simulink subsystem "WinchControl"  (R2022b)
settings: Solver=VariableStepAuto  StartTime=0.0  StopTime=10.0  RelTol=1e-3
undefined symbols (not defined in the file or in its folder): constr, DiscIntNeverNeededParam, params, winchParameter
libraries: simulink x5, slpidlib x1
settings Model: Creator=dylaneijkelhof  LastModifiedBy=jesse
settings SolverCC: AlgebraicLoopSolver=TrustRegion
settings DebuggingCC: UnconnectedInputMsg=warning  UnconnectedOutputMsg=warning  UnconnectedLineMsg=warning  SFMachineParentedDataDiag=warning
settings ModelReferenceCC: EnableRefExpFcnMdlSchedulingChecks=on

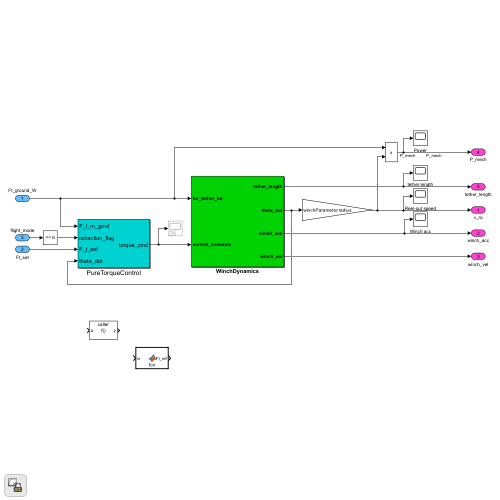
[thumbnail: Simulink's stored preview of the top-level diagram]
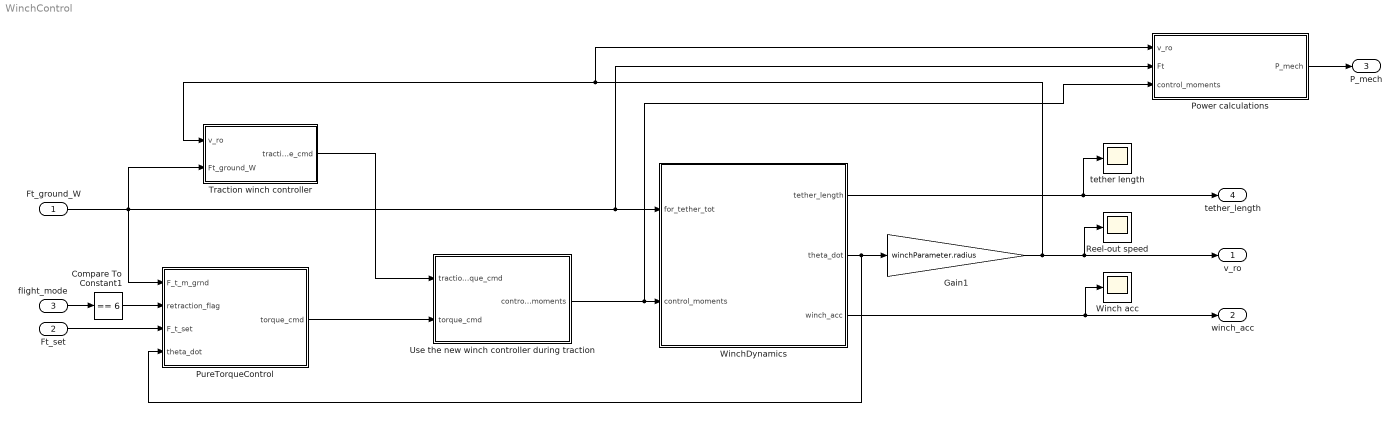
== system WinchControl ==
  Ft_ground_W : Inport  OutDataTypeStr=double  PortDimensions=1
  Ft_set : Inport  Port=2  OutDataTypeStr=double  PortDimensions=1
  flight_mode : Inport  Port=3  OutDataTypeStr=double  PortDimensions=1
  Compare To Constant1 : simulink/Logic and Bit Operations/Compare To Constant  relop===  const=6  OutDataTypeStr=boolean
  Gain1 : Gain  Gain=winchParameter.radius
  Power calculations : Subsystem
  PureTorqueControl : Subsystem
  Reel-out speed : Scope
  Traction winch controller : Subsystem
  Use the new winch controller during traction : Subsystem
  Winch acc : Scope
  WinchDynamics : Subsystem
  tether length : Scope
  v_ro : Outport  OutDataTypeStr=double  PortDimensions=1  VectorParamsAs1DForOutWhenUnconnected=off
  winch_acc : Outport  Port=2  OutDataTypeStr=double  PortDimensions=1  VectorParamsAs1DForOutWhenUnconnected=off
  P_mech : Outport  Port=3  OutDataTypeStr=double  PortDimensions=1  VectorParamsAs1DForOutWhenUnconnected=off
  tether_length : Outport  Port=4  OutDataTypeStr=double  PortDimensions=1  VectorParamsAs1DForOutWhenUnconnected=off
  wires:
  Compare To Constant1/1 -> PureTorqueControl/2(retraction_flag)
  WinchDynamics/1(tether_length) -> tether_length/1, tether length/1
  WinchDynamics/3(winch_acc) -> winch_acc/1, Winch acc/1
  flight_mode/1 -> Compare To Constant1/1
  Ft_set/1 -> PureTorqueControl/3(F_t_set)
  Ft_ground_W/1 -> Power calculations/2(Ft), WinchDynamics/1(for_tether_tot), PureTorqueControl/1(F_t_m_grnd), Traction winch controller/2(Ft_ground_W)
  WinchDynamics/2(theta_dot) -> PureTorqueControl/4(theta_dot), Gain1/1
  Gain1/1 -> Traction winch controller/1(v_ro), Power calculations/1(v_ro), v_ro/1, Reel-out speed/1
  Use the new winch controller during traction/1(control_moments) -> WinchDynamics/2(control_moments), Power calculations/3(control_moments)
  Traction winch controller/1(traction_torque_cmd) -> Use the new winch controller during traction/1(traction_torque_cmd)
  Power calculations/1(P_mech) -> P_mech/1
  PureTorqueControl/1(torque_cmd) -> Use the new winch controller during traction/2(torque_cmd)

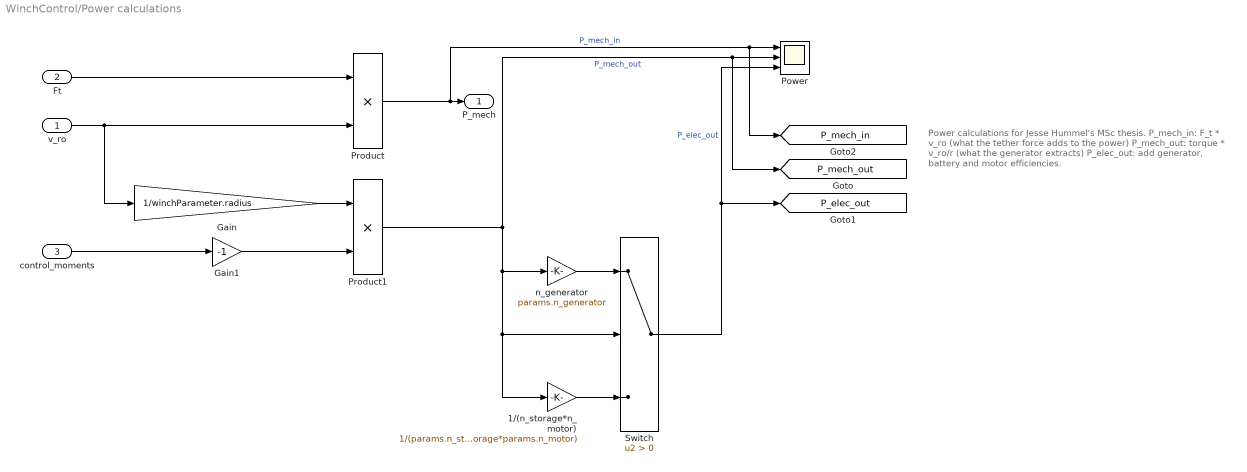
== system WinchControl/Power calculations ==
  note: Power calculations for Jesse Hummel's MSc thesis.
      | P_mech_in: F_t * v_ro (what the tether force adds to the power)
      | P_mech_out: torque * v_ro/r (what the generator extracts)
      | P_elec_out: add generator, battery and motor efficiencies.
  v_ro : Inport
  Ft : Inport  Port=2
  control_moments : Inport  Port=3
  1/(n_storage*n_motor) : Gain  Gain=1/(params.n_storage*params.n_motor)
  Gain : Gain  Gain=1/winchParameter.radius
  Gain1 : Gain  Gain=-1
  Power : Scope  NumInputPorts=3
  Product : Product
  Product1 : Product
  Switch : Switch  Criteria=u2 > Threshold  SaturateOnIntegerOverflow=off  InputSameDT=off
  n_generator : Gain  Gain=params.n_generator
  P_mech : Outport
  tag scope: P_elec_out=global, P_mech_in=global, P_mech_out=global
  wires:
  Gain1/1 -> Product1/2
  Switch/1 -> Power/3, [P_elec_out]  "P_elec_out"
  1/(n_storage*n_motor)/1 -> Switch/3
  n_generator/1 -> Switch/1
  Product1/1 -> Power/2, [P_mech_out], 1/(n_storage*n_motor)/1, Switch/2, n_generator/1  "P_mech_out"
  control_moments/1 -> Gain1/1
  Gain/1 -> Product1/1
  v_ro/1 -> Product/2, Gain/1
  Ft/1 -> Product/1
  Product/1 -> P_mech/1, Power/1, [P_mech_in]  "P_mech_in"

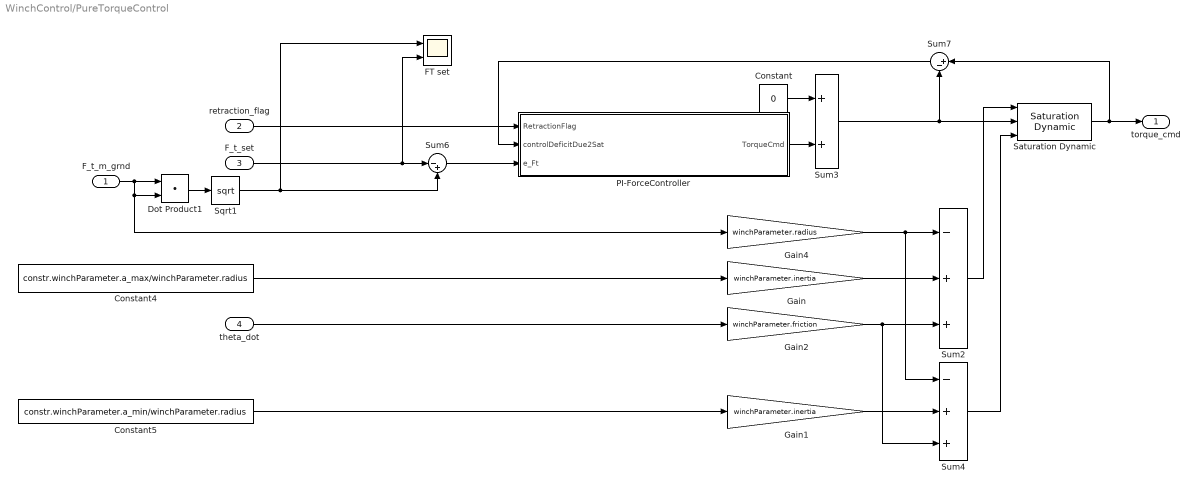
== system WinchControl/PureTorqueControl ==
  F_t_m_grnd : Inport
  retraction_flag : Inport  Port=2
  F_t_set : Inport  Port=3
  theta_dot : Inport  Port=4
  Constant : Constant  Value=0
  Constant4 : Constant  Value=constr.winchParameter.a_max/winchParameter.radius
  Constant5 : Constant  Value=constr.winchParameter.a_min/winchParameter.radius
  Dot Product1 : DotProduct  OutDataTypeStr=Inherit: Inherit via internal rule
  FT set : Scope  NumInputPorts=2
  Gain : Gain  Gain=winchParameter.inertia
  Gain1 : Gain  Gain=winchParameter.inertia
  Gain2 : Gain  Gain=winchParameter.friction
  Gain4 : Gain  Gain=winchParameter.radius
  PI-ForceController : Subsystem
  Saturation Dynamic : simulink/Discontinuities/Saturation Dynamic  OutMin=[]  OutMax=[]  OutDataTypeStr=Inherit: Same as second input  OutDataType=fixdt(1, 16)  OutScaling=2^-10  DoSatur=off
  Sqrt1 : Sqrt
  Sum2 : Sum  Inputs=-++
  Sum3 : Sum
  Sum4 : Sum  Inputs=-++
  Sum6 : Sum  Inputs=|-+
  Sum7 : Sum  Inputs=|+-
  torque_cmd : Outport  VectorParamsAs1DForOutWhenUnconnected=off
  wires:
  Saturation Dynamic/1 -> Sum7/1, torque_cmd/1
  PI-ForceController/1(TorqueCmd) -> Sum3/2
  Sum6/1 -> PI-ForceController/3(e_Ft)
  Sum7/1 -> PI-ForceController/2(controlDeficitDue2Sat)
  theta_dot/1 -> Gain2/1
  F_t_m_grnd/1 -> Gain4/1, Dot Product1/2, Dot Product1/1
  Dot Product1/1 -> Sqrt1/1
  Gain2/1 -> Sum2/3, Sum4/3
  Sum3/1 -> Sum7/2, Saturation Dynamic/2
  Sum4/1 -> Saturation Dynamic/3
  Gain1/1 -> Sum4/2
  Constant5/1 -> Gain1/1
  Sum2/1 -> Saturation Dynamic/1
  Gain/1 -> Sum2/2
  Constant4/1 -> Gain/1
  Gain4/1 -> Sum4/1, Sum2/1
  F_t_set/1 -> Sum6/1, FT set/2
  Constant/1 -> Sum3/1
  retraction_flag/1 -> PI-ForceController/1(RetractionFlag)
  Sqrt1/1 -> Sum6/2, FT set/1

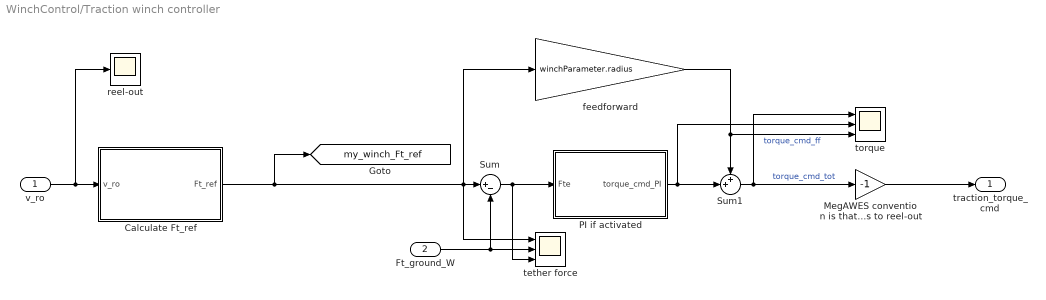
== system WinchControl/Traction winch controller ==
  v_ro : Inport
  Ft_ground_W : Inport  Port=2
  Calculate Ft_ref : Subsystem
  MegAWES convention is that a positive torque leads to reel-out : Gain  Gain=-1
  PI if activated : Subsystem
  Sum : Sum  Inputs=|+-
  Sum1 : Sum  Inputs=++|
  feedforward : Gain  Gain=winchParameter.radius
  reel-out : Scope
  tether force : Scope  NumInputPorts=3
  torque : Scope  NumInputPorts=3
  traction_torque_cmd : Outport
  tag scope: my_winch_Ft_ref=global
  wires:
  PI if activated/1(torque_cmd_PI) -> torque/2, Sum1/2
  Calculate Ft_ref/1(Ft_ref) -> Sum/1, tether force/1, feedforward/1, [my_winch_Ft_ref]
  MegAWES convention is that a positive torque leads to reel-out/1 -> traction_torque_cmd/1
  feedforward/1 -> torque/3, Sum1/1  "torque_cmd_ff"
  Sum1/1 -> torque/1, MegAWES convention is that a positive torque leads to reel-out/1  "torque_cmd_tot"
  Sum/1 -> PI if activated/1(Fte), tether force/3
  Ft_ground_W/1 -> tether force/2, Sum/2
  v_ro/1 -> Calculate Ft_ref/1(v_ro), reel-out/1

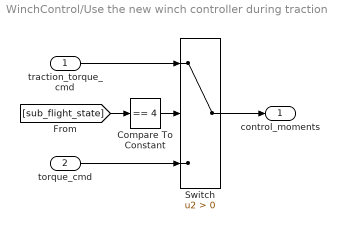
== system WinchControl/Use the new winch controller during traction ==
  traction_torque_cmd : Inport
  torque_cmd : Inport  Port=2
  Compare To Constant : simulink/Logic and Bit Operations/Compare To Constant  relop===  const=4  OutDataTypeStr=boolean
  Switch : Switch  Criteria=u2 > Threshold  SaturateOnIntegerOverflow=off  InputSameDT=off
  control_moments : Outport
  wires:
  Switch/1 -> control_moments/1
  torque_cmd/1 -> Switch/3
  [sub_flight_state] -> Compare To Constant/1
  Compare To Constant/1 -> Switch/2
  traction_torque_cmd/1 -> Switch/1

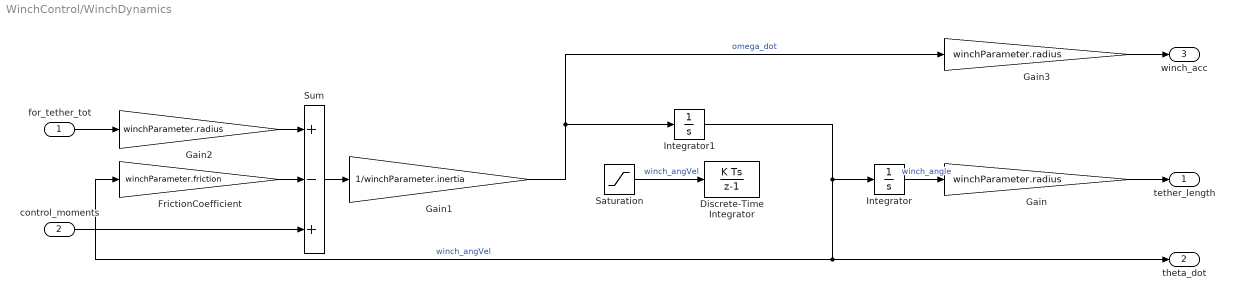
== system WinchControl/WinchDynamics ==
  for_tether_tot : Inport
  control_moments : Inport  Port=2
  Discrete-Time Integrator : DiscreteIntegrator  InitialCondition=winchParameter.lj_dot_init  SampleTime=-1  LimitOutput=on  UpperSaturationLimit=constr.winchParameter.v_max/winchParameter.radius  LowerSaturationLimit=constr.winchParameter.v_min/winchParameter.radius  ICPrevOutput=DiscIntNeverNeededParam  ICPrevScaledInput=DiscIntNeverNeededParam
  FrictionCoefficient : Gain  Gain=winchParameter.friction
  Gain : Gain  Gain=winchParameter.radius
  Gain1 : Gain  Gain=1/winchParameter.inertia
  Gain2 : Gain  Gain=winchParameter.radius
  Gain3 : Gain  Gain=winchParameter.radius
  Integrator : Integrator  InitialCondition=winchParameter.winch_angle_init
  Integrator1 : Integrator
  Saturation : Saturate  UpperLimit=constr.winchParameter.a_max/winchParameter.radius  LowerLimit=constr.winchParameter.a_min/winchParameter.radius
  Sum : Sum  Inputs=+-+
  tether_length : Outport  VectorParamsAs1DForOutWhenUnconnected=off
  theta_dot : Outport  Port=2  VectorParamsAs1DForOutWhenUnconnected=off
  winch_acc : Outport  Port=3  VectorParamsAs1DForOutWhenUnconnected=off
  wires:
  Saturation/1 -> Discrete-Time Integrator/1  "winch_angVel"
  Gain3/1 -> winch_acc/1
  Gain1/1 -> Gain3/1, Integrator1/1  "omega_dot"
  for_tether_tot/1 -> Gain2/1
  FrictionCoefficient/1 -> Sum/2
  control_moments/1 -> Sum/3
  Integrator1/1 -> theta_dot/1, FrictionCoefficient/1, Integrator/1  "winch_angVel"
  Integrator/1 -> Gain/1  "winch_angle"
  Sum/1 -> Gain1/1
  Gain2/1 -> Sum/1
  Gain/1 -> tether_length/1

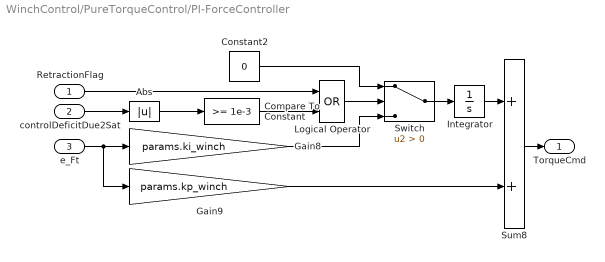
== system WinchControl/PureTorqueControl/PI-ForceController ==
  RetractionFlag : Inport
  controlDeficitDue2Sat : Inport  Port=2
  e_Ft : Inport  Port=3
  Abs : Abs  SaturateOnIntegerOverflow=off
  Compare To Constant : simulink/Logic and Bit Operations/Compare To Constant  relop=>=  const=1e-3  OutDataTypeStr=boolean
  Constant2 : Constant  Value=0
  Gain8 : Gain  Gain=params.ki_winch
  Gain9 : Gain  Gain=params.kp_winch
  Integrator : Integrator
  Logical Operator : Logic  Operator=OR  AllPortsSameDT=off  OutDataTypeStr=boolean
  Sum8 : Sum
  Switch : Switch  Criteria=u2 > Threshold  SaturateOnIntegerOverflow=off  InputSameDT=off
  TorqueCmd : Outport  VectorParamsAs1DForOutWhenUnconnected=off
  wires:
  Logical Operator/1 -> Switch/2
  RetractionFlag/1 -> Logical Operator/1
  controlDeficitDue2Sat/1 -> Abs/1
  e_Ft/1 -> Gain9/1, Gain8/1
  Abs/1 -> Compare To Constant/1
  Integrator/1 -> Sum8/1
  Compare To Constant/1 -> Logical Operator/2
  Gain8/1 -> Switch/3
  Gain9/1 -> Sum8/2
  Constant2/1 -> Switch/1
  Switch/1 -> Integrator/1
  Sum8/1 -> TorqueCmd/1

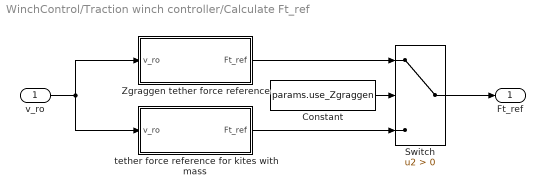
== system WinchControl/Traction winch controller/Calculate Ft_ref ==
  v_ro : Inport
  Constant : Constant  Value=params.use_Zgraggen
  Switch : Switch  Criteria=u2 > Threshold  SaturateOnIntegerOverflow=off  InputSameDT=off
  Zgraggen tether force reference : MATLAB Function  TreatAsAtomicUnit=on
  tether force reference for kites with mass : MATLAB Function  TreatAsAtomicUnit=on
  Ft_ref : Outport
  wires:
  Constant/1 -> Switch/2
  tether force reference for kites with mass/1(Ft_ref) -> Switch/3
  v_ro/1 -> tether force reference for kites with mass/1(v_ro), Zgraggen tether force reference/1(v_ro)
  Switch/1 -> Ft_ref/1
  Zgraggen tether force reference/1(Ft_ref) -> Switch/1

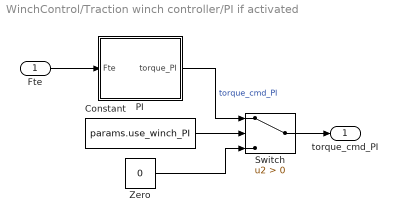
== system WinchControl/Traction winch controller/PI if activated ==
  Fte : Inport
  Constant : Constant  Value=params.use_winch_PI
  PI : Subsystem
  Switch : Switch  Criteria=u2 > Threshold  SaturateOnIntegerOverflow=off  InputSameDT=off
  Zero : Constant  Value=0  OutDataTypeStr=Inherit: Inherit via back propagation
  torque_cmd_PI : Outport
  wires:
  Constant/1 -> Switch/2
  Zero/1 -> Switch/3
  Fte/1 -> PI/1(Fte)
  Switch/1 -> torque_cmd_PI/1
  PI/1(torque_PI) -> Switch/1  "torque_cmd_PI"

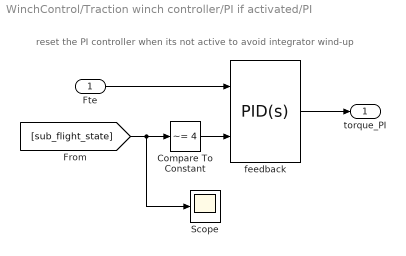
== system WinchControl/Traction winch controller/PI if activated/PI ==
  note: reset the PI controller when its not active to avoid integrator wind-up
  Fte : Inport
  Compare To Constant : simulink/Logic and Bit Operations/Compare To Constant  relop=~=  const=4  OutDataTypeStr=boolean
  Scope : Scope
  feedback : slpidlib/PID Controller  Controller=PID  Form=Parallel  TimeDomain=Continuous-time  UseExternalTs=off  SampleTime=-1  IntegratorMethod=Forward Euler  FilterMethod=Forward Euler  ControllerParametersSource=internal  P=params.kp_traction_winch  I=params.ki_traction_winch  UseKiTs=off  D=0  N=100  UseFilter=on  TunerSelectOption=Transfer Function Based (PID Tuner App)  InitialConditionSource=internal  InitialConditionForIntegrator=0  InitialConditionForFilter=0  DifferentiatorICPrevScaledInput=0  ExternalReset=level  TrackingMode=off  Kt=1  LimitOutput=off  SatLimitsSource=internal  UpperSaturationLimit=inf  LowerSaturationLimit=-inf  LinearizeAsGain=on  AntiWindupMode=none  Kb=1  LimitIntegrator=off  UpperIntegratorSaturationLimit=inf  LowerIntegratorSaturationLimit=-inf  POutMin=[]  POutMax=[]  IOutMin=[]  IOutMax=[]  DOutMin=[]  DOutMax=[]  NOutMin=[]  NOutMax=[]  SumOutMin=[]  SumOutMax=[]  SaturationOutMin=[]  SaturationOutMax=[]  PParamMin=[]  PParamMax=[]  IParamMin=[]  IParamMax=[]  DParamMin=[]  DParamMax=[]  NParamMin=[]  NParamMax=[]  KbParamMin=[]  KbParamMax=[]  KtParamMin=[]  KtParamMax=[]  KbOutMin=[]  KbOutMax=[]  KtOutMin=[]  KtOutMax=[]  IntegratorOutMin=[]  IntegratorOutMax=[]  FilterOutMin=[]  FilterOutMax=[]  SumI1OutMin=[]  SumI1OutMax=[]  SumI2OutMin=[]  SumI2OutMax=[]  SumI3OutMin=[]  SumI3OutMax=[]  SumI4OutMin=[]  SumI4OutMax=[]  SumDOutMin=[]  SumDOutMax=[]  DifferentiatorOutMin=[]  DifferentiatorOutMax=[]  FilterDiffOutCoefMin=[]  FilterDiffOutCoefMax=[]  ReciprocalOutMin=[]  ReciprocalOutMax=[]  SumDenOutMin=[]  SumDenOutMax=[]  SumNumOutMin=[]  SumNumOutMax=[]  DivideOutMin=[]  DivideOutMax=[]  UdiffTsProdOutMin=[]  UdiffTsProdOutMax=[]  NTsProdOutMin=[]  NTsProdOutMax=[]  UintegralTsProdOutMin=[]  UintegralTsProdOutMax=[]  UngainTsProdOutMin=[]  UngainTsProdOutMax=[]  ClampingZeroOutDataTypeStr=Inherit: Inherit via back propagation  ClampingZeroOutMin=[]  ClampingZeroOutMax=[]  FilterDenConstantOutDataTypeStr=Inherit: Inherit via back propagation  FilterDenConstantOutMin=[]  FilterDenConstantOutMax=[]  PCopyOutDataTypeStr=Inherit: Inherit via back propagation  PCopyOutMin=[]  PCopyOutMax=[]  NCopyOutDataTypeStr=Inherit: Inherit via back propagation  NCopyOutMin=[]  NCopyOutMax=[]  IntegratorContinuousStateAttributes=''  IntegratorStateMustResolveToSignalObject=off  IntegratorRTWStateStorageClass=Auto  FilterContinuousStateAttributes=''  FilterStateMustResolveToSignalObject=off  FilterRTWStateStorageClass=Auto  ParallelPVariant=InternalParameters  IdealPVariant=Disabled  IVariant=InternalParameters  DVariant=InternalParameters  IntegratorVariant=Continuous  SatVariant=Disabled  AWVariant=Passthrough  PCopyVariant=Disabled  TRVariant=Disabled  FdbkBlocksVariant=Forward  IdealPFdbkVariant=Disabled  SatFdbkVariant=Disabled  DerivativeFilterVariant=ContFilter  NVariant=InternalParameters  NCopyVariant=Disabled  FilterICVariant=InternalICsFilter  IntegratorICVariant=InternalICs  ExternalResetVariant=ExternalReset  TRSumVariant=Passthrough  SumFdbkVariant=Disabled  SumVariant=Sum_PID  TsampFilterVariant=InternalTs  TsampNgainVariant=Passthrough  TsampIntegralVariant=Passthrough  ExternalSaturationOutDataTypeStr=Inherit: Same as second input
  torque_PI : Outport
  wires:
  feedback/1 -> torque_PI/1
  Fte/1 -> feedback/1
  [sub_flight_state] -> Scope/1, Compare To Constant/1
  Compare To Constant/1 -> feedback/2

== matlab function WinchControl/Traction winch controller/Calculate Ft_ref/Zgraggen tether force reference ==
  data: v_ro input; Ft_ref output; winchParameter parameter; params parameter
function Ft_ref = fcn(v_ro, winchParameter, params)
% From Zgraggen (2016): "Automatic Retraction and Full-Cycle Operation for a
% Class of Airborne Wind Energy Generators".

C = 7.7008e3;  % Hard-coded for the MegAWES kite.
r_m = winchParameter.radius;

if v_ro > 0
    Ft_ref = 4*C*v_ro^2;
else
    Ft_ref = 0.0;
end

% If the winch controls the max tether force, implement a ceiling. + There
% is always a minimum tether force.
winch_controls_max_tether_force = ~params.use_kite_tether_force_control;
if winch_controls_max_tether_force
    Ft_ref = min(max(Ft_ref, params.winch_Ft_min), params.winch_Ft_max);
else
    Ft_ref = max(Ft_ref, params.winch_Ft_min);
end

== matlab function WinchControl/Traction winch controller/Calculate Ft_ref/tether force reference for kites with mass ==
  data: v_ro input; Ft_ref output; params parameter
function Ft_ref = fcn(v_ro, params)
% If the kite is not doing tether force control, the winch should do it.
winch_controls_max_tether_force = ~params.use_kite_tether_force_control;

% This function is just a wrapper around this function.
Ft_ref = Ft_ref_with_mass(v_ro, winch_controls_max_tether_force, ...
    params.winch_Ft_min, params.winch_Ft_max);
